simulink model "MinMax"  (R2020a)
settings: Solver=VariableStepAuto  StartTime=0.0  StopTime=10.0  RelTol=1e-3
settings Model: Creator=royde  LastModifiedBy=royde

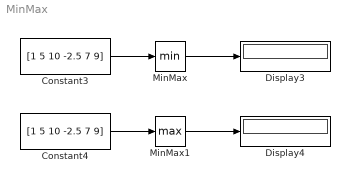
== system MinMax ==
  Constant3 : Constant  Value=[1 5 10 -2.5 7 9]
  Constant4 : Constant  Value=[1 5 10 -2.5 7 9]
  Display3 : Display
  Display4 : Display
  MinMax : MinMax
  MinMax1 : MinMax  Function=max
  wires:
  Constant3/1 -> MinMax/1
  MinMax/1 -> Display3/1
  MinMax1/1 -> Display4/1
  Constant4/1 -> MinMax1/1
